simulink library "ESTS_LSM"  (R2023b)
settings: Solver=VariableStepAuto  StartTime=0.0  StopTime=10.0  RelTol=1e-3
undefined symbols (not defined in the file or in its folder): ESTS_LSM_p_SwitchTime_s, ESTS_LSM_p_TiSample_s
libraries: ESTS_LSM_DEC x1, ESTS_LSM_DYN x1, ESTS_LSM_SM x1, VUT_lib x1
settings Model: Creator=blatak  LastModifiedBy=blatak
settings ModelReferenceCC: EnableRefExpFcnMdlSchedulingChecks=on

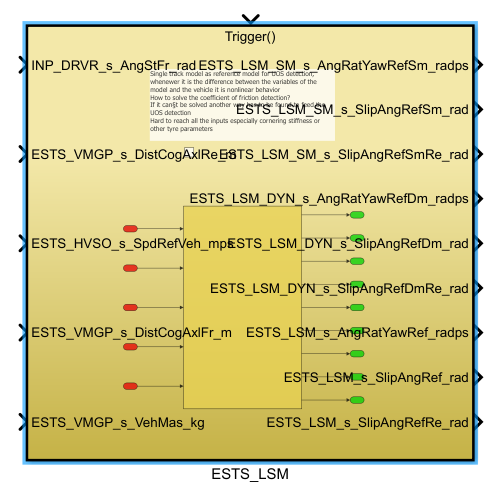
[thumbnail: Simulink's stored preview of the top-level diagram]
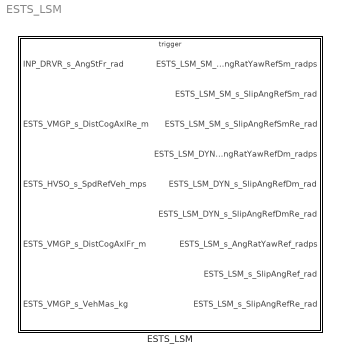
== system ESTS_LSM ==
  ESTS_LSM : Subsystem

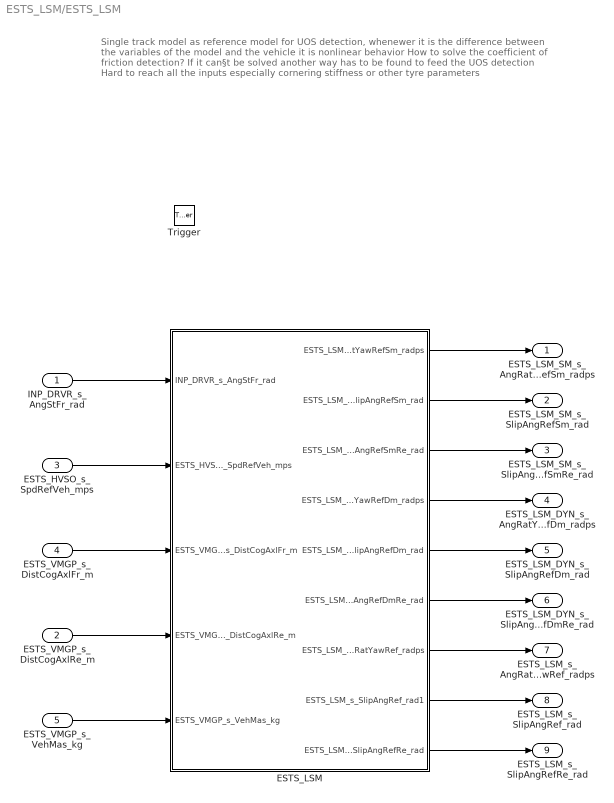
== system ESTS_LSM/ESTS_LSM ==
  note: Single track model as reference model for UOS detection,
      | whenewer it is the difference between the variables of the model and the vehicle it is nonlinear behavior
      | How to solve the coefficient of friction detection?
      | If it can§t be solved another way has to be found to feed the
      | UOS detection
      | Hard to reach all the inputs especially cornering stiffness or other tyre parameters
  INP_DRVR_s_AngStFr_rad : Inport
  ESTS_VMGP_s_DistCogAxlRe_m : Inport  Port=2
  ESTS_HVSO_s_SpdRefVeh_mps : Inport  Port=3
  ESTS_VMGP_s_DistCogAxlFr_m : Inport  Port=4
  ESTS_VMGP_s_VehMas_kg : Inport  Port=5
  Trigger : TriggerPort  TriggerType=function-call  VariantControl=(inherit)  PortDimensions=1
  ESTS_LSM : Subsystem
  ESTS_LSM_SM_s_AngRatYawRefSm_radps : Outport
  ESTS_LSM_SM_s_SlipAngRefSm_rad : Outport  Port=2
  ESTS_LSM_SM_s_SlipAngRefSmRe_rad : Outport  Port=3
  ESTS_LSM_DYN_s_AngRatYawRefDm_radps : Outport  Port=4
  ESTS_LSM_DYN_s_SlipAngRefDm_rad : Outport  Port=5
  ESTS_LSM_DYN_s_SlipAngRefDmRe_rad : Outport  Port=6
  ESTS_LSM_s_AngRatYawRef_radps : Outport  Port=7
  ESTS_LSM_s_SlipAngRef_rad : Outport  Port=8
  ESTS_LSM_s_SlipAngRefRe_rad : Outport  Port=9
  wires:
  INP_DRVR_s_AngStFr_rad/1 -> ESTS_LSM/1(INP_DRVR_s_AngStFr_rad)
  ESTS_LSM/1(ESTS_LSM_SM_s_AngRatYawRefSm_radps) -> ESTS_LSM_SM_s_AngRatYawRefSm_radps/1
  ESTS_LSM/2(ESTS_LSM_SM_s_SlipAngRefSm_rad) -> ESTS_LSM_SM_s_SlipAngRefSm_rad/1
  ESTS_VMGP_s_DistCogAxlFr_m/1 -> ESTS_LSM/3(ESTS_VMGP_s_DistCogAxlFr_m)
  ESTS_HVSO_s_SpdRefVeh_mps/1 -> ESTS_LSM/2(ESTS_HVSO_s_SpdRefVeh_mps)
  ESTS_VMGP_s_VehMas_kg/1 -> ESTS_LSM/5(ESTS_VMGP_s_VehMas_kg)
  ESTS_LSM/3(ESTS_LSM_SM_s_SlipAngRefSmRe_rad) -> ESTS_LSM_SM_s_SlipAngRefSmRe_rad/1
  ESTS_VMGP_s_DistCogAxlRe_m/1 -> ESTS_LSM/4(ESTS_VMGP_s_DistCogAxlRe_m)
  ESTS_LSM/4(ESTS_LSM_DYN_s_AngRatYawRefDm_radps) -> ESTS_LSM_DYN_s_AngRatYawRefDm_radps/1
  ESTS_LSM/5(ESTS_LSM_DYN_s_SlipAngRefDm_rad) -> ESTS_LSM_DYN_s_SlipAngRefDm_rad/1
  ESTS_LSM/6(ESTS_LSM_DYN_s_SlipAngRefDmRe_rad) -> ESTS_LSM_DYN_s_SlipAngRefDmRe_rad/1
  ESTS_LSM/7(ESTS_LSM_s_AngRatYawRef_radps) -> ESTS_LSM_s_AngRatYawRef_radps/1
  ESTS_LSM/8(ESTS_LSM_s_SlipAngRef_rad1) -> ESTS_LSM_s_SlipAngRef_rad/1
  ESTS_LSM/9(ESTS_LSM_s_SlipAngRefRe_rad) -> ESTS_LSM_s_SlipAngRefRe_rad/1

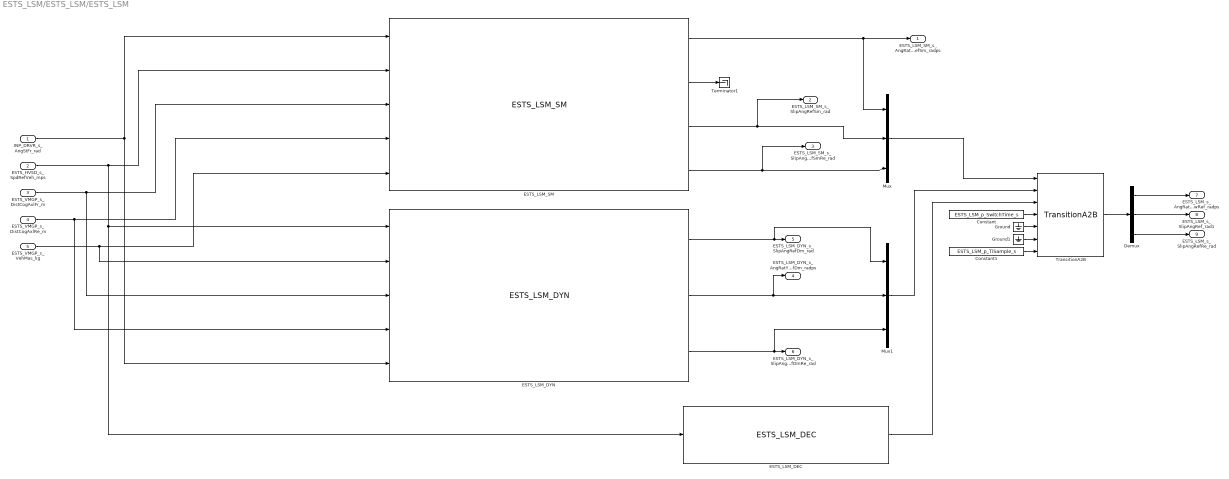
== system ESTS_LSM/ESTS_LSM/ESTS_LSM ==
  INP_DRVR_s_AngStFr_rad : Inport  Description=|
      | Steering wheel angle front - calculated as an average FL and FR,
      | used for single track model, later more sophisticated calculation method needed 
      | than only an average
  ESTS_HVSO_s_SpdRefVeh_mps : Inport  Description=Estimated reference vehicle speed  Port=2
  ESTS_VMGP_s_DistCogAxlFr_m : Inport  Description=X distance from front axle (wheel center) to cog  Port=3
  ESTS_VMGP_s_DistCogAxlRe_m : Inport  Description=X distance from rear axle (wheel center) to cog  Port=4
  ESTS_VMGP_s_VehMas_kg : Inport  Description=Vehicle mass  Port=5
  Constant : Constant  Value=ESTS_LSM_p_SwitchTime_s
  Constant1 : Constant  Description=|  Value=ESTS_LSM_p_TiSample_s
      | Steering wheel angle front - calculated as an average FL and FR,
      | used for single track model, later more sophisticated calculation method needed 
      | than only an average
  Demux : Demux  Outputs=3
  ESTS_LSM_DEC : ESTS_LSM_DEC/ESTS_LSM_DEC  SystemSampleTime=-1  VariantActivationTime=update diagram  AllowFlexibleInterface=on  Latency=0  AutoFrameSizeCalculation=off
  ESTS_LSM_DYN : ESTS_LSM_DYN/ESTS_LSM_DYN  SystemSampleTime=-1  VariantActivationTime=update diagram  AllowFlexibleInterface=on  Latency=0  AutoFrameSizeCalculation=off
  ESTS_LSM_SM : ESTS_LSM_SM/ESTS_LSM_SM  SystemSampleTime=-1  VariantActivationTime=update diagram  AllowFlexibleInterface=on  Latency=0  AutoFrameSizeCalculation=off
  Ground : Ground
  Ground1 : Ground
  Mux : Mux  Inputs=3
  Mux1 : Mux  Inputs=3
  Terminator1 : Terminator
  TransitionA2B : VUT_lib/TransitionA2B  SystemSampleTime=-1  VariantActivationTime=update diagram  AllowFlexibleInterface=on  Latency=0  AutoFrameSizeCalculation=off
  ESTS_LSM_SM_s_AngRatYawRefSm_radps : Outport
  ESTS_LSM_SM_s_SlipAngRefSm_rad : Outport  Port=2
  ESTS_LSM_SM_s_SlipAngRefSmRe_rad : Outport  Port=3
  ESTS_LSM_DYN_s_AngRatYawRefDm_radps : Outport  Port=4
  ESTS_LSM_DYN_s_SlipAngRefDm_rad : Outport  Port=5
  ESTS_LSM_DYN_s_SlipAngRefDmRe_rad : Outport  Port=6
  ESTS_LSM_s_AngRatYawRef_radps : Outport  Description=Reference yaw velocity from single track model  Port=7
  ESTS_LSM_s_SlipAngRef_rad1 : Outport  Description=Reference slip angle in cog from single track model  Port=8
  ESTS_LSM_s_SlipAngRefRe_rad : Outport  Description=Reference slip angle on rear axle from single track model  Port=9
  wires:
  ESTS_LSM_DYN/1 -> Mux1/1, ESTS_LSM_DYN_s_SlipAngRefDm_rad/1
  Mux/1 -> TransitionA2B/1
  Demux/2 -> ESTS_LSM_s_SlipAngRef_rad1/1
  ESTS_LSM_SM/4 -> Mux/3, ESTS_LSM_SM_s_SlipAngRefSmRe_rad/1
  Ground/1 -> TransitionA2B/5
  Mux1/1 -> TransitionA2B/2
  ESTS_LSM_DEC/1 -> TransitionA2B/3
  Ground1/1 -> TransitionA2B/6
  TransitionA2B/1 -> Demux/1
  ESTS_LSM_DYN/3 -> Mux1/3, ESTS_LSM_DYN_s_SlipAngRefDmRe_rad/1
  ESTS_LSM_SM/2 -> Terminator1/1
  Constant1/1 -> TransitionA2B/7
  Demux/1 -> ESTS_LSM_s_AngRatYawRef_radps/1
  Demux/3 -> ESTS_LSM_s_SlipAngRefRe_rad/1
  ESTS_LSM_SM/1 -> ESTS_LSM_SM_s_AngRatYawRefSm_radps/1, Mux/1
  ESTS_LSM_DYN/2 -> Mux1/2, ESTS_LSM_DYN_s_AngRatYawRefDm_radps/1
  ESTS_LSM_SM/3 -> Mux/2, ESTS_LSM_SM_s_SlipAngRefSm_rad/1
  Constant/1 -> TransitionA2B/4
  ESTS_VMGP_s_DistCogAxlFr_m/1 -> ESTS_LSM_DYN/3, ESTS_LSM_SM/3
  INP_DRVR_s_AngStFr_rad/1 -> ESTS_LSM_DYN/5, ESTS_LSM_SM/1
  ESTS_VMGP_s_VehMas_kg/1 -> ESTS_LSM_DYN/2, ESTS_LSM_SM/5
  ESTS_HVSO_s_SpdRefVeh_mps/1 -> ESTS_LSM_SM/2, ESTS_LSM_DEC/1, ESTS_LSM_DYN/1
  ESTS_VMGP_s_DistCogAxlRe_m/1 -> ESTS_LSM_DYN/4, ESTS_LSM_SM/4
